simulink model "Assignment1JM2015a"  (R2015a)
settings: Solver=ode45  StartTime=0.0  StopTime=80  RelTol=1e-3
values from neighbouring files (symbols this model uses):
  Aa0 = 0    [Assignment1JM.m]
  L = Manual_L    (= 9)    [Assignment1JM.m]
  L1 = Manual_L1    (= -1)    [Assignment1JM.m]
  L2 = Manual_L2    (= 6)    [Assignment1JM.m]
  SA = Manual_SA    (= 0)    [Assignment1JM.m]
  v1 = 5    [Assignment1JM.m]
settings Model: Creator=Job  LastModifiedBy=Job

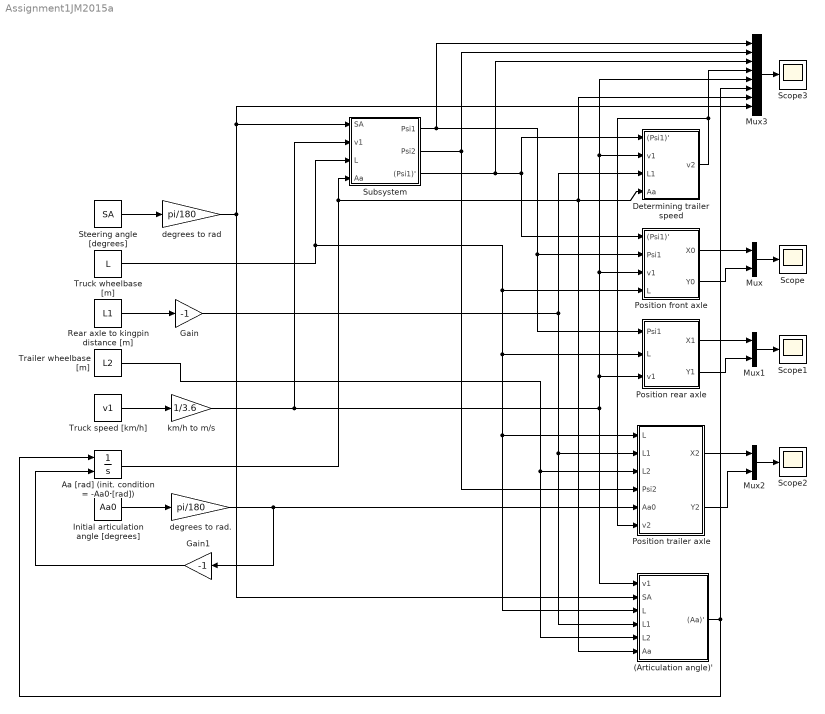
== system Assignment1JM2015a ==
  (Articulation angle)' : Subsystem
  Aa [rad] (init. condition = -Aa0 [rad]) : Integrator  InitialConditionSource=external  InitialCondition=((-Aa0*pi)/180)
  Determining trailer speed : Subsystem
  Gain : Gain  Gain=-1
  Gain1 : Gain  Gain=-1
  Initial articulation angle [degrees] : Constant  Value=Aa0
  Mux : Mux  Inputs=2
  Mux1 : Mux  Inputs=2
  Mux2 : Mux  Inputs=2
  Mux3 : Mux  Inputs=8
  Position front axle : Subsystem
  Position rear axle : Subsystem
  Position trailer axle : Subsystem
  Rear axle to kingpin distance [m] : Constant  Value=L1
  Scope{,1..3} (4 alike) : Scope
      Scope settings: SaveName=DATA0
      Scope1 settings: SaveName=DATA1
      Scope2 settings: SaveName=DATA2
      Scope3 settings: SaveName=DATA3
  Steering angle [degrees] : Constant  Value=SA
  Subsystem : Subsystem
  "Trailer wheelbase [m] " : Constant  Value=L2
  Truck speed [km/h] : Constant  Value=v1
  Truck wheelbase [m] : Constant  Value=L
  degrees to rad : Gain  Gain=pi/180
  degrees to rad. : Gain  Gain=pi/180
  km/h to m/s : Gain  Gain=1/3.6
  wires:
  (Articulation angle)'/1((Aa)') -> Aa [rad] (init. condition = -Aa0 [rad])/1, Mux3/6
  Steering angle [degrees]/1 -> degrees to rad/1
  Truck speed [km/h]/1 -> km/h to m/s/1
  Subsystem/1(Psi1) -> Mux3/1, Position rear axle/1(Psi1), Position front axle/2(Psi1)
  Aa [rad] (init. condition = -Aa0 [rad])/1 -> Mux3/7, Determining trailer speed/4(Aa), (Articulation angle)'/6(Aa), Subsystem/4(Aa)
  Rear axle to kingpin distance [m]/1 -> Gain/1
  "Trailer wheelbase [m] "/1 -> (Articulation angle)'/5(L2), Position trailer axle/3(L2)
  Truck wheelbase [m]/1 -> Subsystem/3(L), Position front axle/4(L), (Articulation angle)'/3(L), Position trailer axle/1(L), Position rear axle/2(L)
  Subsystem/3((Psi1)') -> Mux3/3, Position front axle/1((Psi1)'), Determining trailer speed/1((Psi1)')
  Position front axle/1(X0) -> Mux/1
  Position rear axle/1(X1) -> Mux1/1
  Position trailer axle/1(X2) -> Mux2/1
  Position front axle/2(Y0) -> Mux/2
  Position rear axle/2(Y1) -> Mux1/2
  Position trailer axle/2(Y2) -> Mux2/2
  Mux/1 -> Scope/1
  Mux1/1 -> Scope1/1
  Mux2/1 -> Scope2/1
  degrees to rad/1 -> Mux3/8, Subsystem/1(SA), (Articulation angle)'/2(SA)
  Subsystem/2(Psi2) -> Mux3/2, Position trailer axle/4(Psi2)
  km/h to m/s/1 -> Subsystem/2(v1), (Articulation angle)'/1(v1), Position rear axle/3(v1), Position front axle/3(v1), Mux3/5, Determining trailer speed/2(v1)
  Mux3/1 -> Scope3/1
  Determining trailer speed/1(v2) -> Position trailer axle/6(v2), Mux3/4
  Initial articulation angle [degrees]/1 -> degrees to rad./1
  degrees to rad./1 -> Gain1/1, Position trailer axle/5(Aa0)
  Gain/1 -> Determining trailer speed/3(L1), (Articulation angle)'/4(L1), Position trailer axle/2(L1)
  Gain1/1 -> Aa [rad] (init. condition = -Aa0 [rad])/2

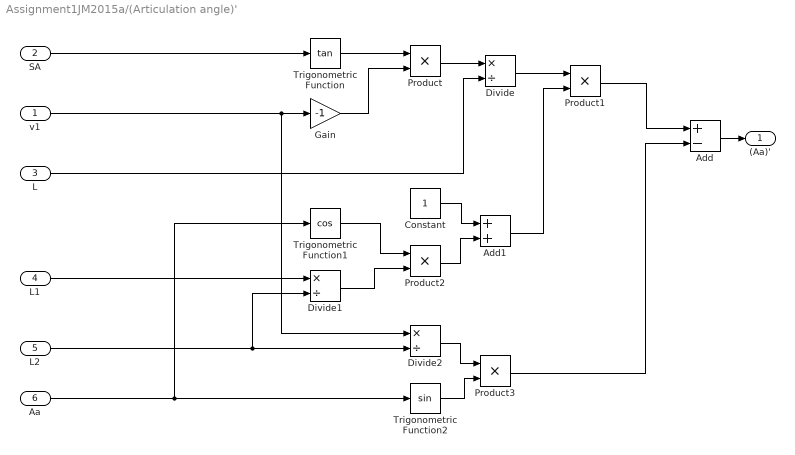
== system Assignment1JM2015a/(Articulation angle)' ==
  v1 : Inport
  SA : Inport  Port=2
  L : Inport  Port=3
  L1 : Inport  Port=4
  L2 : Inport  Port=5
  Aa : Inport  Port=6
  Add : Sum  Inputs=+-
  Add1 : Sum
  Constant : Constant
  Divide : Product  Inputs=*/
  Divide1 : Product  Inputs=*/
  Divide2 : Product  Inputs=*/
  Gain : Gain  Gain=-1
  Product{,1..3} (4 alike) : Product
  Trigonometric Function : Trigonometry  Operator=tan
  Trigonometric Function1 : Trigonometry  Operator=cos
  Trigonometric Function2 : Trigonometry
  (Aa)' : Outport
  wires:
  Trigonometric Function/1 -> Product/1
  Product/1 -> Divide/1
  L/1 -> Divide/2
  SA/1 -> Trigonometric Function/1
  v1/1 -> Divide2/1, Gain/1
  Add/1 -> (Aa)'/1
  Divide/1 -> Product1/1
  Product1/1 -> Add/1
  Constant/1 -> Add1/1
  Product2/1 -> Add1/2
  Trigonometric Function1/1 -> Product2/1
  Divide1/1 -> Product2/2
  Divide2/1 -> Product3/1
  Trigonometric Function2/1 -> Product3/2
  Product3/1 -> Add/2
  Add1/1 -> Product1/2
  Aa/1 -> Trigonometric Function1/1, Trigonometric Function2/1
  L2/1 -> Divide1/2, Divide2/2
  Gain/1 -> Product/2
  L1/1 -> Divide1/1

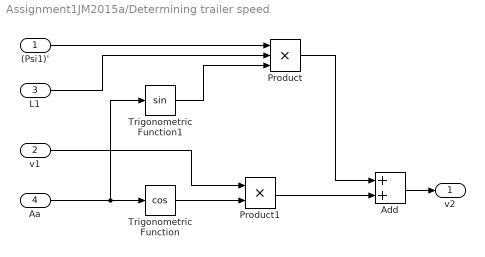
== system Assignment1JM2015a/Determining trailer speed ==
  (Psi1)' : Inport
  v1 : Inport  Port=2
  L1 : Inport  Port=3
  Aa : Inport  Port=4
  Add : Sum
  Product : Product  Inputs=3
  Product1 : Product
  Trigonometric Function : Trigonometry  Operator=cos
  Trigonometric Function1 : Trigonometry
  v2 : Outport
  wires:
  Aa/1 -> Trigonometric Function1/1, Trigonometric Function/1
  Trigonometric Function/1 -> Product1/2
  v1/1 -> Product1/1
  L1/1 -> Product/2
  (Psi1)'/1 -> Product/1
  Add/1 -> v2/1
  Product/1 -> Add/1
  Trigonometric Function1/1 -> Product/3
  Product1/1 -> Add/2

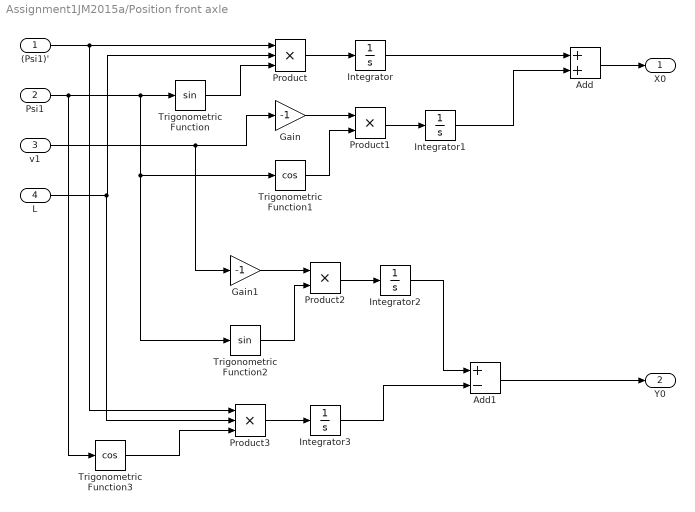
== system Assignment1JM2015a/Position front axle ==
  (Psi1)' : Inport
  Psi1 : Inport  Port=2
  v1 : Inport  Port=3
  L : Inport  Port=4
  Add : Sum
  Add1 : Sum  Inputs=+-
  Gain : Gain  Gain=-1
  Gain1 : Gain  Gain=-1
  Integrator{,1..3} (4 alike) : Integrator
  Product : Product  Inputs=3
  Product1 : Product
  Product2 : Product
  Product3 : Product  Inputs=3
  Trigonometric Function : Trigonometry
  Trigonometric Function1 : Trigonometry  Operator=cos
  Trigonometric Function2 : Trigonometry
  Trigonometric Function3 : Trigonometry  Operator=cos
  X0 : Outport
  Y0 : Outport  Port=2
  wires:
  Psi1/1 -> Trigonometric Function3/1, Trigonometric Function2/1, Trigonometric Function1/1, Trigonometric Function/1
  (Psi1)'/1 -> Product3/1, Product/1
  L/1 -> Product3/2, Product/2
  Trigonometric Function/1 -> Product/3
  Product/1 -> Integrator/1
  Add/1 -> X0/1
  Gain/1 -> Product1/1
  Trigonometric Function1/1 -> Product1/2
  Product1/1 -> Integrator1/1
  Integrator1/1 -> Add/2
  Integrator/1 -> Add/1
  v1/1 -> Gain1/1, Gain/1
  Gain1/1 -> Product2/1
  Trigonometric Function2/1 -> Product2/2
  Product2/1 -> Integrator2/1
  Trigonometric Function3/1 -> Product3/3
  Product3/1 -> Integrator3/1
  Integrator3/1 -> Add1/2
  Integrator2/1 -> Add1/1
  Add1/1 -> Y0/1

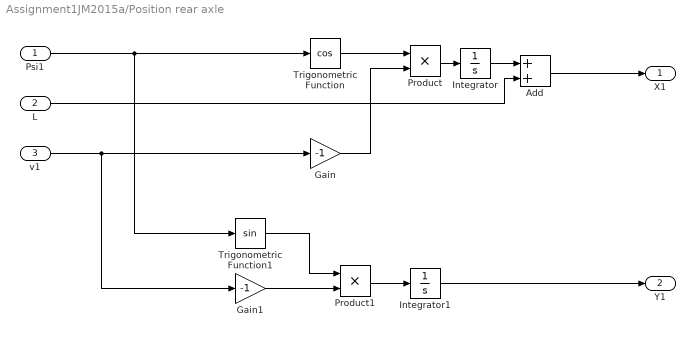
== system Assignment1JM2015a/Position rear axle ==
  Psi1 : Inport
  L : Inport  Port=2
  v1 : Inport  Port=3
  Add : Sum
  Gain : Gain  Gain=-1
  Gain1 : Gain  Gain=-1
  Integrator : Integrator
  Integrator1 : Integrator
  Product : Product
  Product1 : Product
  Trigonometric Function : Trigonometry  Operator=cos
  Trigonometric Function1 : Trigonometry
  X1 : Outport
  Y1 : Outport  Port=2
  wires:
  Psi1/1 -> Trigonometric Function1/1, Trigonometric Function/1
  v1/1 -> Gain1/1, Gain/1
  Trigonometric Function/1 -> Product/1
  Gain/1 -> Product/2
  Product/1 -> Integrator/1
  L/1 -> Add/2
  Add/1 -> X1/1
  Integrator/1 -> Add/1
  Gain1/1 -> Product1/2
  Trigonometric Function1/1 -> Product1/1
  Product1/1 -> Integrator1/1
  Integrator1/1 -> Y1/1

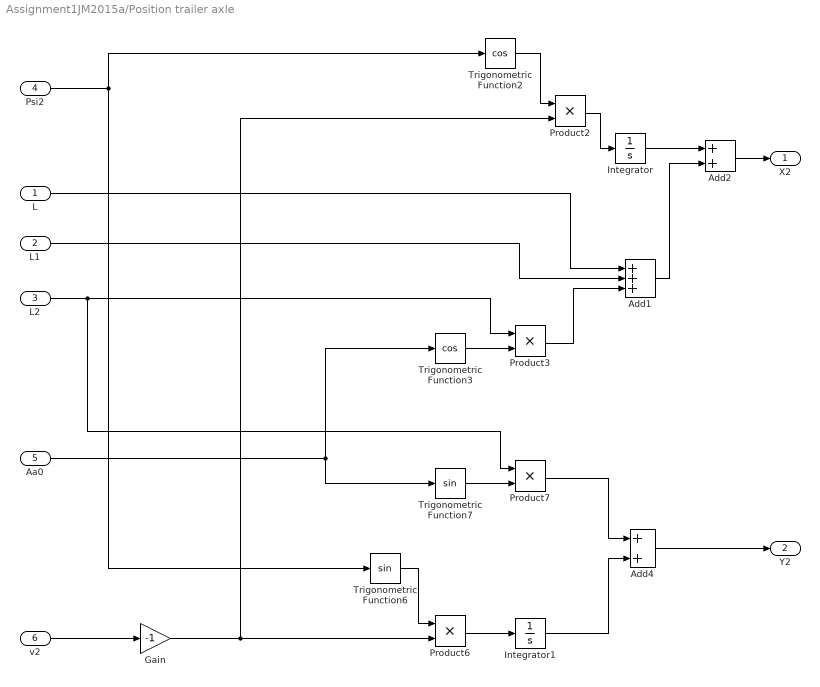
== system Assignment1JM2015a/Position trailer axle ==
  L : Inport
  L1 : Inport  Port=2
  L2 : Inport  Port=3
  Psi2 : Inport  Port=4
  Aa0 : Inport  Port=5
  v2 : Inport  Port=6
  Add1 : Sum  Inputs=+++
  Add2 : Sum
  Add4 : Sum
  Gain : Gain  Gain=-1
  Integrator : Integrator
  Integrator1 : Integrator
  Product{2..3,6..7} (4 alike) : Product
  Trigonometric Function2 : Trigonometry  Operator=cos
  Trigonometric Function3 : Trigonometry  Operator=cos
  Trigonometric Function6 : Trigonometry
  Trigonometric Function7 : Trigonometry
  X2 : Outport
  Y2 : Outport  Port=2
  wires:
  L/1 -> Add1/1
  Trigonometric Function2/1 -> Product2/1
  Product2/1 -> Integrator/1
  Aa0/1 -> Trigonometric Function3/1, Trigonometric Function7/1
  Trigonometric Function3/1 -> Product3/2
  L2/1 -> Product7/1, Product3/1
  Product3/1 -> Add1/3
  Integrator/1 -> Add2/1
  Add2/1 -> X2/1
  Add1/1 -> Add2/2
  Trigonometric Function6/1 -> Product6/1
  Trigonometric Function7/1 -> Product7/2
  Add4/1 -> Y2/1
  Integrator1/1 -> Add4/2
  Product7/1 -> Add4/1
  L1/1 -> Add1/2
  Product6/1 -> Integrator1/1
  Psi2/1 -> Trigonometric Function6/1, Trigonometric Function2/1
  v2/1 -> Gain/1
  Gain/1 -> Product2/2, Product6/2

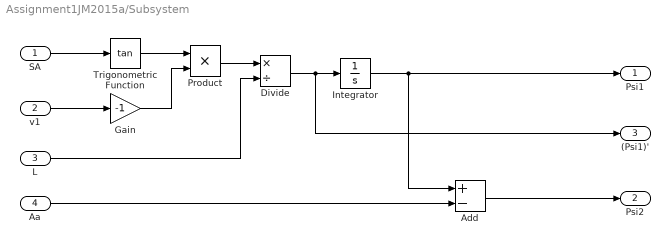
== system Assignment1JM2015a/Subsystem ==
  SA : Inport
  v1 : Inport  Port=2
  L : Inport  Port=3
  Aa : Inport  Port=4
  Add : Sum  Inputs=+-
  Divide : Product  Inputs=*/
  Gain : Gain  Gain=-1
  Integrator : Integrator
  Product : Product
  Trigonometric Function : Trigonometry  Operator=tan
  Psi1 : Outport
  Psi2 : Outport  Port=2
  (Psi1)' : Outport  Port=3
  wires:
  SA/1 -> Trigonometric Function/1
  v1/1 -> Gain/1
  Trigonometric Function/1 -> Product/1
  Gain/1 -> Product/2
  Product/1 -> Divide/1
  L/1 -> Divide/2
  Divide/1 -> (Psi1)'/1, Integrator/1
  Aa/1 -> Add/2
  Integrator/1 -> Add/1, Psi1/1
  Add/1 -> Psi2/1
